simulink model "pendulo_filtro"  (R2020b)
settings: Solver=FixedStepAuto  StartTime=0.0  StopTime=10  FixedStep=1e-3  RelTol=1e-3
values from neighbouring files (symbols this model uses):
  controlador = projetarControlador(requisitos, planta)    [executarTudo.m]    (also in runAll.m)
  model = obterParametros(planta, varianciaComando, varianciaMedida)    [executarTudo.m]    (also in runAll.m)
  planta = obterPlanta()    [codetest.m]    (also in executarTudo.m; nextState.m; runAll.m)
  thetar = 0    [executarTudo.m]    (also in runAll.m)
undefined symbols (not defined in the file or in its folder): varCom, varMed
libraries: pid_lib x1
settings Model: Creator=davi  LastModifiedBy=alvar

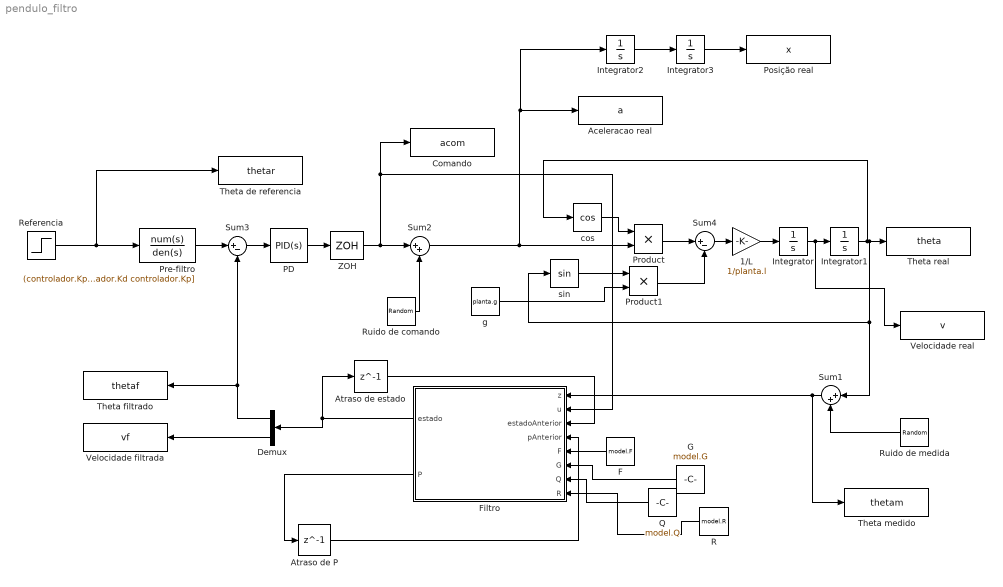
== system pendulo_filtro ==
  1/L : Gain  Gain=1/planta.l
  Aceleracao real : ToWorkspace  VariableName=a  SaveFormat=Structure With Time  SampleTime=-1
  Atraso de P : Delay  DelayLength=1  InitialCondition=eye(2)  SampleTime=model.T
  Atraso de estado : Delay  DelayLength=1  InitialCondition=[0;0]  SampleTime=model.T
  Comando : ToWorkspace  VariableName=acom  SaveFormat=Structure With Time  SampleTime=-1
  Demux : Demux  Outputs=2
  F : Constant  Value=model.F
  Filtro : MATLAB Function  TreatAsAtomicUnit=on  SystemSampleTime=1e-2
  G : Constant  Value=model.G
  Integrator{,1..3} (4 alike) : Integrator
  PD : pid_lib/PID Controller  Controller=PID  Form=Parallel  TimeDomain=Continuous-time  UseExternalTs=off  SampleTime=1e-2  IntegratorMethod=Forward Euler  FilterMethod=Forward Euler  ControllerParametersSource=internal  P=controlador.Kp  I=0  D=controlador.Kd  UseFilter=on  N=100  TunerSelectOption=Transfer Function Based (PID Tuner App)  InitialConditionSource=internal  InitialConditionForIntegrator=0  InitialConditionForFilter=0  DifferentiatorICPrevScaledInput=0  ExternalReset=none  TrackingMode=off  Kt=1  LimitOutput=off  SatLimitsSource=internal  UpperSaturationLimit=inf  LowerSaturationLimit=-inf  LinearizeAsGain=on  AntiWindupMode=none  Kb=1  POutMin=[]  POutMax=[]  IOutMin=[]  IOutMax=[]  DOutMin=[]  DOutMax=[]  NOutMin=[]  NOutMax=[]  SumOutMin=[]  SumOutMax=[]  SaturationOutMin=[]  SaturationOutMax=[]  PParamMin=[]  PParamMax=[]  IParamMin=[]  IParamMax=[]  DParamMin=[]  DParamMax=[]  NParamMin=[]  NParamMax=[]  KbParamMin=[]  KbParamMax=[]  KtParamMin=[]  KtParamMax=[]  KbOutMin=[]  KbOutMax=[]  KtOutMin=[]  KtOutMax=[]  IntegratorOutMin=[]  IntegratorOutMax=[]  FilterOutMin=[]  FilterOutMax=[]  SumI1OutMin=[]  SumI1OutMax=[]  SumI2OutMin=[]  SumI2OutMax=[]  SumI3OutMin=[]  SumI3OutMax=[]  SumI4OutMin=[]  SumI4OutMax=[]  SumDOutMin=[]  SumDOutMax=[]  DifferentiatorOutMin=[]  DifferentiatorOutMax=[]  FilterDiffOutCoefMin=[]  FilterDiffOutCoefMax=[]  ReciprocalOutMin=[]  ReciprocalOutMax=[]  SumDenOutMin=[]  SumDenOutMax=[]  SumNumOutMin=[]  SumNumOutMax=[]  DivideOutMin=[]  DivideOutMax=[]  UdiffTsProdOutMin=[]  UdiffTsProdOutMax=[]  NTsProdOutMin=[]  NTsProdOutMax=[]  UintegralTsProdOutMin=[]  UintegralTsProdOutMax=[]  UngainTsProdOutMin=[]  UngainTsProdOutMax=[]  IntegratorContinuousStateAttributes=''  IntegratorStateMustResolveToSignalObject=off  IntegratorRTWStateStorageClass=Auto  FilterContinuousStateAttributes=''  FilterStateMustResolveToSignalObject=off  FilterRTWStateStorageClass=Auto  ParallelPVariant=InternalParameters  IdealPVariant=Disabled  IVariant=InternalParameters  DVariant=InternalParameters  IntegratorVariant=Continuous  SatVariant=Disabled  AWVariant=Passthrough  PCopyVariant=Disabled  TRVariant=Disabled  FdbkBlocksVariant=Forward  IdealPFdbkVariant=Disabled  SatFdbkVariant=Disabled  DerivativeFilterVariant=ContFilter  NVariant=InternalParameters  NCopyVariant=Disabled  FilterICVariant=InternalICsFilter  IntegratorICVariant=InternalICs  ExternalResetVariant=Disabled  TRSumVariant=Passthrough  SumFdbkVariant=Disabled  SumVariant=Sum_PID  TsampFilterVariant=InternalTs  TsampNgainVariant=Passthrough  TsampIntegralVariant=Passthrough  ExternalSaturationOutDataTypeStr=Inherit: Same as second input
  Posição real : ToWorkspace  VariableName=x  SaveFormat=Structure With Time  SampleTime=-1
  Pre-filtro : TransferFcn  Numerator=(controlador.Kp+planta.g)  Denominator=[controlador.Kd controlador.Kp]
  Product : Product
  Product1 : Product
  Q : Constant  Value=model.Q
  R : Constant  Value=model.R
  Referencia : Step  Time=0  After=thetar  SampleTime=0
  Ruido de comando : RandomNumber  Variance=varCom  SampleTime=1e-2
  Ruido de medida : RandomNumber  Variance=varMed  SampleTime=1e-2
  Sum1 : Sum  Inputs=|++
  Sum2 : Sum  Inputs=|++
  Sum3 : Sum  Inputs=|+-
  Sum4 : Sum  Inputs=|+-
  Theta de referencia : ToWorkspace  VariableName=thetar  SaveFormat=Structure With Time  SampleTime=-1
  Theta filtrado : ToWorkspace  VariableName=thetaf  SaveFormat=Structure With Time  SampleTime=-1
  Theta medido : ToWorkspace  VariableName=thetam  SaveFormat=Structure With Time  SampleTime=-1
  Theta real : ToWorkspace  VariableName=theta  SaveFormat=Structure With Time  SampleTime=-1
  Velocidade filtrada : ToWorkspace  VariableName=vf  SaveFormat=Structure With Time  SampleTime=-1
  Velocidade real : ToWorkspace  VariableName=v  SaveFormat=Structure With Time  SampleTime=-1
  ZOH : ZeroOrderHold  SampleTime=model.T
  cos : Trigonometry  Operator=cos
  g : Constant  Value=planta.g
  sin : Trigonometry
  wires:
  Product/1 -> Sum4/1
  Ruido de medida/1 -> Sum1/2
  Ruido de comando/1 -> Sum2/2
  Referencia/1 -> Pre-filtro/1, Theta de referencia/1
  Pre-filtro/1 -> Sum3/1
  cos/1 -> Product/1
  sin/1 -> Product1/1
  g/1 -> Product1/2
  Product1/1 -> Sum4/2
  Sum4/1 -> 1/L/1
  1/L/1 -> Integrator/1
  Integrator/1 -> Velocidade real/1, Integrator1/1
  Integrator1/1 -> sin/1, Sum1/1, Theta real/1, cos/1
  Sum3/1 -> PD/1
  Sum1/1 -> Theta medido/1, Filtro/1(z)
  Filtro/1(estado) -> Atraso de estado/1, Demux/1
  Filtro/2(P) -> Atraso de P/1
  Atraso de estado/1 -> Filtro/3(estadoAnterior)
  Atraso de P/1 -> Filtro/4(pAnterior)
  Demux/2 -> Velocidade filtrada/1
  Demux/1 -> Sum3/2, Theta filtrado/1
  PD/1 -> ZOH/1
  ZOH/1 -> Filtro/2(u), Comando/1, Sum2/1
  F/1 -> Filtro/5(F)
  G/1 -> Filtro/6(G)
  Q/1 -> Filtro/7(Q)
  R/1 -> Filtro/8(R)
  Sum2/1 -> Product/2, Integrator2/1, Aceleracao real/1
  Integrator2/1 -> Integrator3/1
  Integrator3/1 -> Posição real/1

== matlab function pendulo_filtro/Filtro ==
  settings: updateMethod=DISCRETE
  data: estado output; z input; u input; estadoAnterior input; pAnterior input; P output; F input; G input; Q input; R input
function [estado, P] = fcn(z, u, estadoAnterior, pAnterior, F, G, Q, R)
% Calcula o estado atual e a matriz de covariância de estado
% Entradas
% z: observação
% u: comando
% F : matriz de transição de estado
% G : matriz de entrada de controle 
% Q : covariância do ruído de movimento
% R : covariância do ruído de medida
% Saidas
% estado: estado atual
% P: matriz de covariância de estado

xPredito = F*estadoAnterior + G*u;
pPredito = F*pAnterior*F' + Q;

C = [1 0];
Kt = pPredito * C' * pinv(R + C*pPredito*C');
estado = xPredito + Kt*(z-C*estadoAnterior);
P = pPredito - Kt*C*pPredito;
end
